simulink model "kurtosis"  (R2012b)
settings: Solver=ode45  StartTime=0.0  StopTime=3171  RelTol=1e-3
libraries: xbsIndex_r4 x3174, casper_library_flow_control x64, casper_library_misc x1, simulink_xsg_bridge x1
(part 4 of 24)

== system kurtosis/multi_to_workspace_complex/to_workspace_cplx_2 ==
  X_fi2 : Inport
  c_to_ri : Subsystem
  imag_gateway : xbsIndex_r4/Gateway Out  inherit_from_input=on  hdl_port=off  timing_constraint=None  locs_specified=off  LOCs={}  UseAsDAC=off  DACChannel='1'  block_type=gatewayout
  real_gateway : xbsIndex_r4/Gateway Out  inherit_from_input=on  hdl_port=off  timing_constraint=None  locs_specified=off  LOCs={}  UseAsDAC=off  DACChannel='1'  block_type=gatewayout
  ri_to_c : RealImagToComplex
  workspace_output : ToWorkspace  VariableName=X_fi2  SampleTime=-1
  _o : Outport
  wires:
  X_fi2/1 -> c_to_ri/1(c), _o/1
  ri_to_c/1 -> workspace_output/1  "cplx"
  imag_gateway/1 -> ri_to_c/2
  real_gateway/1 -> ri_to_c/1
  c_to_ri/2(im) -> imag_gateway/1  "c_to_ri_out2"
  c_to_ri/1(re) -> real_gateway/1  "c_to_ri_out1"

== system kurtosis/multi_to_workspace_complex/to_workspace_cplx_3 ==
  X_fi3 : Inport
  c_to_ri : Subsystem
  imag_gateway : xbsIndex_r4/Gateway Out  inherit_from_input=on  hdl_port=off  timing_constraint=None  locs_specified=off  LOCs={}  UseAsDAC=off  DACChannel='1'  block_type=gatewayout
  real_gateway : xbsIndex_r4/Gateway Out  inherit_from_input=on  hdl_port=off  timing_constraint=None  locs_specified=off  LOCs={}  UseAsDAC=off  DACChannel='1'  block_type=gatewayout
  ri_to_c : RealImagToComplex
  workspace_output : ToWorkspace  VariableName=X_fi3  SampleTime=-1
  _o : Outport
  wires:
  X_fi3/1 -> c_to_ri/1(c), _o/1
  ri_to_c/1 -> workspace_output/1  "cplx"
  imag_gateway/1 -> ri_to_c/2
  real_gateway/1 -> ri_to_c/1
  c_to_ri/2(im) -> imag_gateway/1  "c_to_ri_out2"
  c_to_ri/1(re) -> real_gateway/1  "c_to_ri_out1"

== system kurtosis/multi_to_workspace_complex/to_workspace_cplx_4 ==
  X_fi4 : Inport
  c_to_ri : Subsystem
  imag_gateway : xbsIndex_r4/Gateway Out  inherit_from_input=on  hdl_port=off  timing_constraint=None  locs_specified=off  LOCs={}  UseAsDAC=off  DACChannel='1'  block_type=gatewayout
  real_gateway : xbsIndex_r4/Gateway Out  inherit_from_input=on  hdl_port=off  timing_constraint=None  locs_specified=off  LOCs={}  UseAsDAC=off  DACChannel='1'  block_type=gatewayout
  ri_to_c : RealImagToComplex
  workspace_output : ToWorkspace  VariableName=X_fi4  SampleTime=-1
  _o : Outport
  wires:
  X_fi4/1 -> c_to_ri/1(c), _o/1
  ri_to_c/1 -> workspace_output/1  "cplx"
  imag_gateway/1 -> ri_to_c/2
  real_gateway/1 -> ri_to_c/1
  c_to_ri/2(im) -> imag_gateway/1  "c_to_ri_out2"
  c_to_ri/1(re) -> real_gateway/1  "c_to_ri_out1"

== system kurtosis/multi_to_workspace_complex/to_workspace_cplx_5 ==
  X_fi5 : Inport
  c_to_ri : Subsystem
  imag_gateway : xbsIndex_r4/Gateway Out  inherit_from_input=on  hdl_port=off  timing_constraint=None  locs_specified=off  LOCs={}  UseAsDAC=off  DACChannel='1'  block_type=gatewayout
  real_gateway : xbsIndex_r4/Gateway Out  inherit_from_input=on  hdl_port=off  timing_constraint=None  locs_specified=off  LOCs={}  UseAsDAC=off  DACChannel='1'  block_type=gatewayout
  ri_to_c : RealImagToComplex
  workspace_output : ToWorkspace  VariableName=X_fi5  SampleTime=-1
  _o : Outport
  wires:
  X_fi5/1 -> c_to_ri/1(c), _o/1
  ri_to_c/1 -> workspace_output/1  "cplx"
  imag_gateway/1 -> ri_to_c/2
  real_gateway/1 -> ri_to_c/1
  c_to_ri/2(im) -> imag_gateway/1  "c_to_ri_out2"
  c_to_ri/1(re) -> real_gateway/1  "c_to_ri_out1"

== system kurtosis/multi_to_workspace_complex/to_workspace_cplx_6 ==
  X_fi6 : Inport
  c_to_ri : Subsystem
  imag_gateway : xbsIndex_r4/Gateway Out  inherit_from_input=on  hdl_port=off  timing_constraint=None  locs_specified=off  LOCs={}  UseAsDAC=off  DACChannel='1'  block_type=gatewayout
  real_gateway : xbsIndex_r4/Gateway Out  inherit_from_input=on  hdl_port=off  timing_constraint=None  locs_specified=off  LOCs={}  UseAsDAC=off  DACChannel='1'  block_type=gatewayout
  ri_to_c : RealImagToComplex
  workspace_output : ToWorkspace  VariableName=X_fi6  SampleTime=-1
  _o : Outport
  wires:
  X_fi6/1 -> c_to_ri/1(c), _o/1
  ri_to_c/1 -> workspace_output/1  "cplx"
  imag_gateway/1 -> ri_to_c/2
  real_gateway/1 -> ri_to_c/1
  c_to_ri/2(im) -> imag_gateway/1  "c_to_ri_out2"
  c_to_ri/1(re) -> real_gateway/1  "c_to_ri_out1"

== system kurtosis/multi_to_workspace_complex/to_workspace_cplx_7 ==
  X_fi7 : Inport
  c_to_ri : Subsystem
  imag_gateway : xbsIndex_r4/Gateway Out  inherit_from_input=on  hdl_port=off  timing_constraint=None  locs_specified=off  LOCs={}  UseAsDAC=off  DACChannel='1'  block_type=gatewayout
  real_gateway : xbsIndex_r4/Gateway Out  inherit_from_input=on  hdl_port=off  timing_constraint=None  locs_specified=off  LOCs={}  UseAsDAC=off  DACChannel='1'  block_type=gatewayout
  ri_to_c : RealImagToComplex
  workspace_output : ToWorkspace  VariableName=X_fi7  SampleTime=-1
  _o : Outport
  wires:
  X_fi7/1 -> c_to_ri/1(c), _o/1
  ri_to_c/1 -> workspace_output/1  "cplx"
  imag_gateway/1 -> ri_to_c/2
  real_gateway/1 -> ri_to_c/1
  c_to_ri/2(im) -> imag_gateway/1  "c_to_ri_out2"
  c_to_ri/1(re) -> real_gateway/1  "c_to_ri_out1"

== system kurtosis/multi_to_workspace_complex/to_workspace_cplx_8 ==
  X_fi8 : Inport
  c_to_ri : Subsystem
  imag_gateway : xbsIndex_r4/Gateway Out  inherit_from_input=on  hdl_port=off  timing_constraint=None  locs_specified=off  LOCs={}  UseAsDAC=off  DACChannel='1'  block_type=gatewayout
  real_gateway : xbsIndex_r4/Gateway Out  inherit_from_input=on  hdl_port=off  timing_constraint=None  locs_specified=off  LOCs={}  UseAsDAC=off  DACChannel='1'  block_type=gatewayout
  ri_to_c : RealImagToComplex
  workspace_output : ToWorkspace  VariableName=X_fi8  SampleTime=-1
  _o : Outport
  wires:
  X_fi8/1 -> c_to_ri/1(c), _o/1
  ri_to_c/1 -> workspace_output/1  "cplx"
  imag_gateway/1 -> ri_to_c/2
  real_gateway/1 -> ri_to_c/1
  c_to_ri/2(im) -> imag_gateway/1  "c_to_ri_out2"
  c_to_ri/1(re) -> real_gateway/1  "c_to_ri_out1"

== system kurtosis/kurtosis/absx_4th_im_ser/par_to_ser ==
  pin : Inport
  ld : Inport  Port=2
  shift : Inport  Port=3
  Logical : xbsIndex_r4/Logical  logical_function=OR  inputs=2  en=off  latency=0  precision=Full  arith_type=Unsigned  n_bits=16  bin_pt=0  align_bp=on  dbl_ovrd=off  block_type=logical
  filler : xbsIndex_r4/Constant  const=0  gui_display_data_type=Fixed-point  arith_type=Unsigned  n_bits=sout_width  bin_pt=0  preci_type=Single  exp_width=8  frac_width=24  explicit_period=on  period=1  equ=P=C  opselect=C  inp2=PCIN>>17  opr=+  inp1=P  carry=CIN  dbl_ovrd=off  block_type=constant
  shifter_unit1 : casper_library_flow_control/shifter_unit  data_width=84  pin_offset=0
  shifter_unit2 : casper_library_flow_control/shifter_unit  data_width=84  pin_offset=84
  shifter_unit3 : casper_library_flow_control/shifter_unit  data_width=84  pin_offset=168
  shifter_unit4 : casper_library_flow_control/shifter_unit  data_width=84  pin_offset=252
  shifter_unit5 : casper_library_flow_control/shifter_unit  data_width=84  pin_offset=336
  shifter_unit6 : casper_library_flow_control/shifter_unit  data_width=84  pin_offset=420
  shifter_unit7 : casper_library_flow_control/shifter_unit  data_width=84  pin_offset=504
  shifter_unit8 : casper_library_flow_control/shifter_unit  data_width=84  pin_offset=588
  sout : Outport
  wires:
  ld/1 -> Logical/1, shifter_unit1/1, shifter_unit2/1, shifter_unit3/1, shifter_unit4/1, shifter_unit5/1, shifter_unit6/1, shifter_unit7/1, shifter_unit8/1
  shift/1 -> Logical/2
  filler/1 -> shifter_unit1/2
  pin/1 -> shifter_unit1/3, shifter_unit2/3, shifter_unit3/3, shifter_unit4/3, shifter_unit5/3, shifter_unit6/3, shifter_unit7/3, shifter_unit8/3
  Logical/1 -> shifter_unit1/4, shifter_unit2/4, shifter_unit3/4, shifter_unit4/4, shifter_unit5/4, shifter_unit6/4, shifter_unit7/4, shifter_unit8/4
  shifter_unit1/1 -> shifter_unit2/2
  shifter_unit2/1 -> shifter_unit3/2
  shifter_unit3/1 -> shifter_unit4/2
  shifter_unit4/1 -> shifter_unit5/2
  shifter_unit5/1 -> shifter_unit6/2
  shifter_unit6/1 -> shifter_unit7/2
  shifter_unit7/1 -> shifter_unit8/2
  shifter_unit8/1 -> sout/1

== system kurtosis/kurtosis/absx_4th_im_ser/pin_concat ==
  in0 : Inport
  in1 : Inport  Port=2
  in2 : Inport  Port=3
  in3 : Inport  Port=4
  in4 : Inport  Port=5
  in5 : Inport  Port=6
  in6 : Inport  Port=7
  in7 : Inport  Port=8
  concat : xbsIndex_r4/Concat  num_inputs=8  dbl_ovrd=off  block_type=concat
  reinterpret_{1..8} (8 alike) : xbsIndex_r4/Reinterpret  force_arith_type=on  arith_type=Unsigned  force_bin_pt=on  bin_pt=0  block_type=reinterpret
  out : Outport
  wires:
  concat/1 -> out/1
  reinterpret_8/1 -> concat/8
  reinterpret_7/1 -> concat/7
  reinterpret_6/1 -> concat/6
  reinterpret_5/1 -> concat/5
  reinterpret_4/1 -> concat/4
  reinterpret_3/1 -> concat/3
  reinterpret_2/1 -> concat/2
  reinterpret_1/1 -> concat/1
  in7/1 -> reinterpret_8/1
  in6/1 -> reinterpret_7/1
  in5/1 -> reinterpret_6/1
  in4/1 -> reinterpret_5/1
  in3/1 -> reinterpret_4/1
  in2/1 -> reinterpret_3/1
  in1/1 -> reinterpret_2/1
  in0/1 -> reinterpret_1/1

== system kurtosis/kurtosis/absx_4th_im_ser/pulse_ext ==
  ld : Inport
  Constant10 : xbsIndex_r4/Constant  const=8  gui_display_data_type=Fixed-point  arith_type=Unsigned  n_bits=4  bin_pt=0  preci_type=Single  exp_width=8  frac_width=24  explicit_period=on  period=1  equ=P=C  opselect=C  inp2=PCIN>>17  opr=+  inp1=P  carry=CIN  dbl_ovrd=off  block_type=constant
  Constant8 : xbsIndex_r4/Constant  const=15  gui_display_data_type=Fixed-point  arith_type=Unsigned  n_bits=4  bin_pt=0  preci_type=Single  exp_width=8  frac_width=24  explicit_period=on  period=1  equ=P=C  opselect=C  inp2=PCIN>>17  opr=+  inp1=P  carry=CIN  dbl_ovrd=off  block_type=constant
  Constant9 : xbsIndex_r4/Constant  const=1  gui_display_data_type=Fixed-point  arith_type=Unsigned  n_bits=4  bin_pt=0  preci_type=Single  exp_width=8  frac_width=24  explicit_period=on  period=1  equ=P=C  opselect=C  inp2=PCIN>>17  opr=+  inp1=P  carry=CIN  dbl_ovrd=off  block_type=constant
  Counter : xbsIndex_r4/Counter  cnt_type=Free Running  cnt_to=Inf  operation=Up  start_count=0  cnt_by_val=1  arith_type=Unsigned  n_bits=4  bin_pt=0  load_pin=off  rst=on  en=on  explicit_period=on  period=1  dbl_ovrd=off  use_behavioral_HDL=off  implementation=Fabric  block_type=counter
  Relational : xbsIndex_r4/Relational  mode=a<b  en=off  latency=0  dbl_ovrd=off  block_type=relational
  Relational1 : xbsIndex_r4/Relational  mode=a<=b  en=off  latency=0  dbl_ovrd=off  block_type=relational
  Relational2 : xbsIndex_r4/Relational  mode=a>=b  en=off  latency=0  dbl_ovrd=off  block_type=relational
  and : xbsIndex_r4/Logical  logical_function=AND  inputs=2  en=off  latency=0  precision=Full  arith_type=Unsigned  n_bits=16  bin_pt=0  align_bp=on  dbl_ovrd=off  block_type=logical
  or : xbsIndex_r4/Logical  logical_function=OR  inputs=2  en=off  latency=0  precision=Full  arith_type=Unsigned  n_bits=16  bin_pt=0  align_bp=on  dbl_ovrd=off  block_type=logical
  shift : Outport
  wires:
  ld/1 -> Counter/1, or/1
  Counter/1 -> Relational2/1, Relational1/1, Relational/1  "Counter_out1"
  Relational2/1 -> and/1  "Relational2_out1"
  Constant9/1 -> Relational2/2
  Relational1/1 -> and/2  "Relational1_out1"
  Constant10/1 -> Relational1/2
  Relational/1 -> or/2  "Relational_out1"
  Constant8/1 -> Relational/2
  and/1 -> shift/1
  or/1 -> Counter/2

== system kurtosis/kurtosis/absx_sq_re_ser/par_to_ser ==
  pin : Inport
  ld : Inport  Port=2
  shift : Inport  Port=3
  Logical : xbsIndex_r4/Logical  logical_function=OR  inputs=2  en=off  latency=0  precision=Full  arith_type=Unsigned  n_bits=16  bin_pt=0  align_bp=on  dbl_ovrd=off  block_type=logical
  filler : xbsIndex_r4/Constant  const=0  gui_display_data_type=Fixed-point  arith_type=Unsigned  n_bits=sout_width  bin_pt=0  preci_type=Single  exp_width=8  frac_width=24  explicit_period=on  period=1  equ=P=C  opselect=C  inp2=PCIN>>17  opr=+  inp1=P  carry=CIN  dbl_ovrd=off  block_type=constant
  shifter_unit1 : casper_library_flow_control/shifter_unit  data_width=35  pin_offset=0
  shifter_unit2 : casper_library_flow_control/shifter_unit  data_width=35  pin_offset=35
  shifter_unit3 : casper_library_flow_control/shifter_unit  data_width=35  pin_offset=70
  shifter_unit4 : casper_library_flow_control/shifter_unit  data_width=35  pin_offset=105
  shifter_unit5 : casper_library_flow_control/shifter_unit  data_width=35  pin_offset=140
  shifter_unit6 : casper_library_flow_control/shifter_unit  data_width=35  pin_offset=175
  shifter_unit7 : casper_library_flow_control/shifter_unit  data_width=35  pin_offset=210
  shifter_unit8 : casper_library_flow_control/shifter_unit  data_width=35  pin_offset=245
  sout : Outport
  wires:
  ld/1 -> Logical/1, shifter_unit1/1, shifter_unit2/1, shifter_unit3/1, shifter_unit4/1, shifter_unit5/1, shifter_unit6/1, shifter_unit7/1, shifter_unit8/1
  shift/1 -> Logical/2
  filler/1 -> shifter_unit1/2
  pin/1 -> shifter_unit1/3, shifter_unit2/3, shifter_unit3/3, shifter_unit4/3, shifter_unit5/3, shifter_unit6/3, shifter_unit7/3, shifter_unit8/3
  Logical/1 -> shifter_unit1/4, shifter_unit2/4, shifter_unit3/4, shifter_unit4/4, shifter_unit5/4, shifter_unit6/4, shifter_unit7/4, shifter_unit8/4
  shifter_unit1/1 -> shifter_unit2/2
  shifter_unit2/1 -> shifter_unit3/2
  shifter_unit3/1 -> shifter_unit4/2
  shifter_unit4/1 -> shifter_unit5/2
  shifter_unit5/1 -> shifter_unit6/2
  shifter_unit6/1 -> shifter_unit7/2
  shifter_unit7/1 -> shifter_unit8/2
  shifter_unit8/1 -> sout/1

== system kurtosis/kurtosis/absx_sq_re_ser/pin_concat ==
  in0 : Inport
  in1 : Inport  Port=2
  in2 : Inport  Port=3
  in3 : Inport  Port=4
  in4 : Inport  Port=5
  in5 : Inport  Port=6
  in6 : Inport  Port=7
  in7 : Inport  Port=8
  concat : xbsIndex_r4/Concat  num_inputs=8  dbl_ovrd=off  block_type=concat
  reinterpret_{1..8} (8 alike) : xbsIndex_r4/Reinterpret  force_arith_type=on  arith_type=Unsigned  force_bin_pt=on  bin_pt=0  block_type=reinterpret
  out : Outport
  wires:
  concat/1 -> out/1
  reinterpret_8/1 -> concat/8
  reinterpret_7/1 -> concat/7
  reinterpret_6/1 -> concat/6
  reinterpret_5/1 -> concat/5
  reinterpret_4/1 -> concat/4
  reinterpret_3/1 -> concat/3
  reinterpret_2/1 -> concat/2
  reinterpret_1/1 -> concat/1
  in7/1 -> reinterpret_8/1
  in6/1 -> reinterpret_7/1
  in5/1 -> reinterpret_6/1
  in4/1 -> reinterpret_5/1
  in3/1 -> reinterpret_4/1
  in2/1 -> reinterpret_3/1
  in1/1 -> reinterpret_2/1
  in0/1 -> reinterpret_1/1

== system kurtosis/kurtosis/absx_sq_re_ser/pulse_ext ==
  ld : Inport
  Constant10 : xbsIndex_r4/Constant  const=8  gui_display_data_type=Fixed-point  arith_type=Unsigned  n_bits=4  bin_pt=0  preci_type=Single  exp_width=8  frac_width=24  explicit_period=on  period=1  equ=P=C  opselect=C  inp2=PCIN>>17  opr=+  inp1=P  carry=CIN  dbl_ovrd=off  block_type=constant
  Constant8 : xbsIndex_r4/Constant  const=15  gui_display_data_type=Fixed-point  arith_type=Unsigned  n_bits=4  bin_pt=0  preci_type=Single  exp_width=8  frac_width=24  explicit_period=on  period=1  equ=P=C  opselect=C  inp2=PCIN>>17  opr=+  inp1=P  carry=CIN  dbl_ovrd=off  block_type=constant
  Constant9 : xbsIndex_r4/Constant  const=1  gui_display_data_type=Fixed-point  arith_type=Unsigned  n_bits=4  bin_pt=0  preci_type=Single  exp_width=8  frac_width=24  explicit_period=on  period=1  equ=P=C  opselect=C  inp2=PCIN>>17  opr=+  inp1=P  carry=CIN  dbl_ovrd=off  block_type=constant
  Counter : xbsIndex_r4/Counter  cnt_type=Free Running  cnt_to=Inf  operation=Up  start_count=0  cnt_by_val=1  arith_type=Unsigned  n_bits=4  bin_pt=0  load_pin=off  rst=on  en=on  explicit_period=on  period=1  dbl_ovrd=off  use_behavioral_HDL=off  implementation=Fabric  block_type=counter
  Relational : xbsIndex_r4/Relational  mode=a<b  en=off  latency=0  dbl_ovrd=off  block_type=relational
  Relational1 : xbsIndex_r4/Relational  mode=a<=b  en=off  latency=0  dbl_ovrd=off  block_type=relational
  Relational2 : xbsIndex_r4/Relational  mode=a>=b  en=off  latency=0  dbl_ovrd=off  block_type=relational
  and : xbsIndex_r4/Logical  logical_function=AND  inputs=2  en=off  latency=0  precision=Full  arith_type=Unsigned  n_bits=16  bin_pt=0  align_bp=on  dbl_ovrd=off  block_type=logical
  or : xbsIndex_r4/Logical  logical_function=OR  inputs=2  en=off  latency=0  precision=Full  arith_type=Unsigned  n_bits=16  bin_pt=0  align_bp=on  dbl_ovrd=off  block_type=logical
  shift : Outport
  wires:
  ld/1 -> Counter/1, or/1
  Counter/1 -> Relational2/1, Relational1/1, Relational/1  "Counter_out1"
  Relational2/1 -> and/1  "Relational2_out1"
  Constant9/1 -> Relational2/2
  Relational1/1 -> and/2  "Relational1_out1"
  Constant10/1 -> Relational1/2
  Relational/1 -> or/2  "Relational_out1"
  Constant8/1 -> Relational/2
  and/1 -> shift/1
  or/1 -> Counter/2

== system kurtosis/kurtosis/kurtosis_acc_bank_1/abs_x_4th_acc ==
  sync : Inport
  b : Inport  Port=2
  Convert : xbsIndex_r4/Convert  gui_display_data_type=Fixed-point  arith_type="Signed  (2's comp)"  n_bits=96  bin_pt=68  float_type=Single  exp_bits=8  fraction_bits=24  quantization=Truncate  overflow=Wrap  en=off  latency=0  dbl_ovrd=off  pipeline=off  block_type=convert
  DSP48E_0 : xbsIndex_r4/DSP48E  use_a=Direct from A Port  use_b=Direct from B Port  reset_preg=off  pattern_from_creg=on  pattern='000000000000'  mask_from_creg=on  pattern_mask='000000000000'  sel_rounding_mask=Select mask  use_op=off  use_creg=on  rst_all=off  en_all=off  use_pcin=off  use_carrycascin=off  use_multsignin=off  use_carryout=on  use_patterndetect=off  use_patternbdetect=off  use_overflow=off  use_underflow=off  use_acout=off  use_bcout=off  use_pcout=off  use_multsignout=off  use_carrycascout=off  pipeline_a=1  pipeline_b=1  pipeline_acout=1  pipeline_bcout=1  pipeline_c=on  pipeline_p=on  pipeline_mult=on  pipeline_opmode=on  pipeline_alumode=on  pipeline_carryin=on  pipeline_carryinsel=on  rst_a=off  rst_b=off  rst_c=off  rst_mult=off  rst_p=off  rst_carry_in=off  rst_alumode=off  rst_ctrl=off  en_a1=off  en_a2=off  en_b1=off  en_b2=off  en_c=off  en_mult=off  en_p=off  en_carry_in=off  en_alumode=off  en_multcarryin=off  en_ctrl=off  use_synth_model=off  addsub_mode=ONE48  xl_useadderonly=off  block_type=dsp48e
  DSP48E_1 : xbsIndex_r4/DSP48E  use_a=Direct from A Port  use_b=Direct from B Port  reset_preg=off  pattern_from_creg=on  pattern='000000000000'  mask_from_creg=on  pattern_mask='000000000000'  sel_rounding_mask=Select mask  use_op=off  use_creg=off  rst_all=off  en_all=off  use_pcin=off  use_carrycascin=off  use_multsignin=off  use_carryout=off  use_patterndetect=off  use_patternbdetect=off  use_overflow=off  use_underflow=off  use_acout=off  use_bcout=off  use_pcout=off  use_multsignout=off  use_carrycascout=off  pipeline_a=2  pipeline_b=2  pipeline_acout=1  pipeline_bcout=1  pipeline_c=on  pipeline_p=on  pipeline_mult=on  pipeline_opmode=on  pipeline_alumode=on  pipeline_carryin=off  pipeline_carryinsel=on  rst_a=off  rst_b=off  rst_c=off  rst_mult=off  rst_p=off  rst_carry_in=off  rst_alumode=off  rst_ctrl=off  en_a1=off  en_a2=off  en_b1=off  en_b2=off  en_c=off  en_mult=off  en_p=off  en_carry_in=off  en_alumode=off  en_multcarryin=off  en_ctrl=off  use_synth_model=off  addsub_mode=ONE48  xl_useadderonly=off  block_type=dsp48e
  DSP48_AB_splitter1 : Subsystem
  DSP48_AB_splitter2_sub : Subsystem
  Delay1 : xbsIndex_r4/Delay  rst=off  infoeditControl=Selection of Reset will increase slice count due to use of real FFs and instead of SRLs  en=off  latency=1  dbl_ovrd=off  reg_retiming=off  block_type=delay
  Mux : xbsIndex_r4/Mux  inputs=2  en=off  latency=0  precision=Full  arith_type=Unsigned  n_bits=16  bin_pt=14  quantization=Truncate  overflow=Wrap  dbl_ovrd=off  block_type=mux
  Mux1 : xbsIndex_r4/Mux  inputs=2  en=off  latency=0  precision=Full  arith_type=Unsigned  n_bits=16  bin_pt=14  quantization=Truncate  overflow=Wrap  dbl_ovrd=off  block_type=mux
  Register : xbsIndex_r4/Register  init=0  rst=off  en=off  dbl_ovrd=off  block_type=register
  Reinterpret : xbsIndex_r4/Reinterpret  force_arith_type=on  arith_type="Signed  (2's comp)"  force_bin_pt=on  bin_pt=0  block_type=reinterpret
  Reinterpret1 : xbsIndex_r4/Reinterpret  force_arith_type=on  arith_type="Signed  (2's comp)"  force_bin_pt=on  bin_pt=0  block_type=reinterpret
  Reinterpret2 : xbsIndex_r4/Reinterpret  force_arith_type=on  arith_type="Signed  (2's comp)"  force_bin_pt=on  bin_pt=68  block_type=reinterpret
  Slice : xbsIndex_r4/Slice  nbits=48  boolean_output=off  mode=Lower Bit Location + Width  bit1=0  base1=MSB of Input  bit0=0  base0=LSB of Input  dbl_ovrd=off  block_type=slice
  Slice2 : xbsIndex_r4/Slice  nbits=48  boolean_output=off  mode=Lower Bit Location + Width  bit1=0  base1=MSB of Input  bit0=48  base0=LSB of Input  dbl_ovrd=off  block_type=slice
  cram : Subsystem
  dsp48e_ctrl_init_xblock14 : Subsystem
  dsp48e_ctrl_init_xblock15 : Subsystem
  opmode_0_rst : xbsIndex_r4/Constant  const=12  gui_display_data_type=Fixed-point  arith_type=Unsigned  n_bits=7  bin_pt=0  preci_type=Single  exp_width=8  frac_width=24  explicit_period=on  period=1  equ=P=C  opselect=C  inp2=PCIN>>17  opr=+  inp1=P  carry=CIN  dbl_ovrd=off  block_type=constant
  opmode_1_rst : xbsIndex_r4/Constant  const=3  gui_display_data_type=Fixed-point  arith_type=Unsigned  n_bits=7  bin_pt=0  preci_type=Single  exp_width=8  frac_width=24  explicit_period=on  period=1  equ=P=C  opselect=C  inp2=PCIN>>17  opr=+  inp1=P  carry=CIN  dbl_ovrd=off  block_type=constant
  zero : xbsIndex_r4/Constant  const=0  gui_display_data_type=Fixed-point  arith_type=Signed (2's comp)  n_bits=48  bin_pt=0  preci_type=Single  exp_width=8  frac_width=24  explicit_period=on  period=1  equ=P=C  opselect=C  inp2=PCIN>>17  opr=+  inp1=P  carry=CIN  dbl_ovrd=off  block_type=constant
  +=b : Outport
  wires:
  sync/1 -> Mux1/1, Mux/1
  Reinterpret1/1 -> Slice2/1, Slice/1  "Reinterpret1_out1"
  dsp48e_ctrl_init_xblock15/4(carryinsel) -> DSP48E_1/6  "dsp48e_ctrl1_out4"
  dsp48e_ctrl_init_xblock15/2(alumode) -> DSP48E_1/4  "dsp48e_ctrl1_out2"
  dsp48e_ctrl_init_xblock15/1(opmode) -> Mux1/2  "dsp48e_ctrl1_out1"
  dsp48e_ctrl_init_xblock14/4(carryinsel) -> DSP48E_0/7  "dsp48e_ctrl0_out4"
  dsp48e_ctrl_init_xblock14/3(carryin) -> DSP48E_0/6  "dsp48e_ctrl0_out3"
  dsp48e_ctrl_init_xblock14/2(alumode) -> DSP48E_0/5  "dsp48e_ctrl0_out2"
  dsp48e_ctrl_init_xblock14/1(opmode) -> Mux/2  "dsp48e_ctrl0_out1"
  DSP48_AB_splitter2_sub/2(B) -> DSP48E_1/2  "DSP48_AB_splitter2_out2"
  DSP48_AB_splitter2_sub/1(A) -> DSP48E_1/1  "DSP48_AB_splitter2_out1"
  Slice2/1 -> DSP48_AB_splitter2_sub/1(A:B)  "Slice2_out1"
  zero/1 -> DSP48_AB_splitter1/1(A:B)  "zero_out1"
  opmode_1_rst/1 -> Mux1/3  "opmode_1_rst_out1"
  opmode_0_rst/1 -> Mux/3  "opmode_0_rst_out1"
  cram/1(Out) -> Reinterpret2/1  "cram_out1"
  Register/1 -> cram/2(In2)  "Register_out1"
  DSP48E_1/1 -> cram/1(In1)  "DSP48E_1_out1"
  Slice/1 -> Reinterpret/1  "Slice_out1"
  Reinterpret2/1 -> +=b/1
  Convert/1 -> Reinterpret1/1  "Convert_out1"
  Reinterpret/1 -> DSP48E_0/3  "Reinterpret_out1"
  DSP48E_0/1 -> Register/1  "DSP48E_0_out1"
  Mux1/1 -> Delay1/1  "Mux1_out1"
  Mux/1 -> DSP48E_0/4  "Mux_out1"
  Delay1/1 -> DSP48E_1/3  "Delay1_out1"
  DSP48_AB_splitter1/2(B) -> DSP48E_0/2  "DSP48_AB_splitter1_out2"
  DSP48_AB_splitter1/1(A) -> DSP48E_0/1  "DSP48_AB_splitter1_out1"
  DSP48E_0/2 -> DSP48E_1/5  "DSP48E_0_out2"
  b/1 -> Convert/1

== system kurtosis/kurtosis/kurtosis_acc_bank_1/abs_x_sq_acc ==
  sync : Inport
  b : Inport  Port=2
  Convert : xbsIndex_r4/Convert  gui_display_data_type=Fixed-point  arith_type="Signed  (2's comp)"  n_bits=96  bin_pt=34  float_type=Single  exp_bits=8  fraction_bits=24  quantization=Truncate  overflow=Wrap  en=off  latency=0  dbl_ovrd=off  pipeline=off  block_type=convert
  DSP48E_0 : xbsIndex_r4/DSP48E  use_a=Direct from A Port  use_b=Direct from B Port  reset_preg=off  pattern_from_creg=on  pattern='000000000000'  mask_from_creg=on  pattern_mask='000000000000'  sel_rounding_mask=Select mask  use_op=off  use_creg=on  rst_all=off  en_all=off  use_pcin=off  use_carrycascin=off  use_multsignin=off  use_carryout=on  use_patterndetect=off  use_patternbdetect=off  use_overflow=off  use_underflow=off  use_acout=off  use_bcout=off  use_pcout=off  use_multsignout=off  use_carrycascout=off  pipeline_a=1  pipeline_b=1  pipeline_acout=1  pipeline_bcout=1  pipeline_c=on  pipeline_p=on  pipeline_mult=on  pipeline_opmode=on  pipeline_alumode=on  pipeline_carryin=on  pipeline_carryinsel=on  rst_a=off  rst_b=off  rst_c=off  rst_mult=off  rst_p=off  rst_carry_in=off  rst_alumode=off  rst_ctrl=off  en_a1=off  en_a2=off  en_b1=off  en_b2=off  en_c=off  en_mult=off  en_p=off  en_carry_in=off  en_alumode=off  en_multcarryin=off  en_ctrl=off  use_synth_model=off  addsub_mode=ONE48  xl_useadderonly=off  block_type=dsp48e
  DSP48E_1 : xbsIndex_r4/DSP48E  use_a=Direct from A Port  use_b=Direct from B Port  reset_preg=off  pattern_from_creg=on  pattern='000000000000'  mask_from_creg=on  pattern_mask='000000000000'  sel_rounding_mask=Select mask  use_op=off  use_creg=off  rst_all=off  en_all=off  use_pcin=off  use_carrycascin=off  use_multsignin=off  use_carryout=off  use_patterndetect=off  use_patternbdetect=off  use_overflow=off  use_underflow=off  use_acout=off  use_bcout=off  use_pcout=off  use_multsignout=off  use_carrycascout=off  pipeline_a=2  pipeline_b=2  pipeline_acout=1  pipeline_bcout=1  pipeline_c=on  pipeline_p=on  pipeline_mult=on  pipeline_opmode=on  pipeline_alumode=on  pipeline_carryin=off  pipeline_carryinsel=on  rst_a=off  rst_b=off  rst_c=off  rst_mult=off  rst_p=off  rst_carry_in=off  rst_alumode=off  rst_ctrl=off  en_a1=off  en_a2=off  en_b1=off  en_b2=off  en_c=off  en_mult=off  en_p=off  en_carry_in=off  en_alumode=off  en_multcarryin=off  en_ctrl=off  use_synth_model=off  addsub_mode=ONE48  xl_useadderonly=off  block_type=dsp48e
  DSP48_AB_splitter1 : Subsystem
  DSP48_AB_splitter2_sub : Subsystem
  Delay1 : xbsIndex_r4/Delay  rst=off  infoeditControl=Selection of Reset will increase slice count due to use of real FFs and instead of SRLs  en=off  latency=1  dbl_ovrd=off  reg_retiming=off  block_type=delay
  Mux : xbsIndex_r4/Mux  inputs=2  en=off  latency=0  precision=Full  arith_type=Unsigned  n_bits=16  bin_pt=14  quantization=Truncate  overflow=Wrap  dbl_ovrd=off  block_type=mux
  Mux1 : xbsIndex_r4/Mux  inputs=2  en=off  latency=0  precision=Full  arith_type=Unsigned  n_bits=16  bin_pt=14  quantization=Truncate  overflow=Wrap  dbl_ovrd=off  block_type=mux
  Register : xbsIndex_r4/Register  init=0  rst=off  en=off  dbl_ovrd=off  block_type=register
  Reinterpret : xbsIndex_r4/Reinterpret  force_arith_type=on  arith_type="Signed  (2's comp)"  force_bin_pt=on  bin_pt=0  block_type=reinterpret
  Reinterpret1 : xbsIndex_r4/Reinterpret  force_arith_type=on  arith_type="Signed  (2's comp)"  force_bin_pt=on  bin_pt=0  block_type=reinterpret
  Reinterpret2 : xbsIndex_r4/Reinterpret  force_arith_type=on  arith_type="Signed  (2's comp)"  force_bin_pt=on  bin_pt=34  block_type=reinterpret
  Slice : xbsIndex_r4/Slice  nbits=48  boolean_output=off  mode=Lower Bit Location + Width  bit1=0  base1=MSB of Input  bit0=0  base0=LSB of Input  dbl_ovrd=off  block_type=slice
  Slice2 : xbsIndex_r4/Slice  nbits=48  boolean_output=off  mode=Lower Bit Location + Width  bit1=0  base1=MSB of Input  bit0=48  base0=LSB of Input  dbl_ovrd=off  block_type=slice
  cram : Subsystem
  dsp48e_ctrl_init_xblock12 : Subsystem
  dsp48e_ctrl_init_xblock13 : Subsystem
  opmode_0_rst : xbsIndex_r4/Constant  const=12  gui_display_data_type=Fixed-point  arith_type=Unsigned  n_bits=7  bin_pt=0  preci_type=Single  exp_width=8  frac_width=24  explicit_period=on  period=1  equ=P=C  opselect=C  inp2=PCIN>>17  opr=+  inp1=P  carry=CIN  dbl_ovrd=off  block_type=constant
  opmode_1_rst : xbsIndex_r4/Constant  const=3  gui_display_data_type=Fixed-point  arith_type=Unsigned  n_bits=7  bin_pt=0  preci_type=Single  exp_width=8  frac_width=24  explicit_period=on  period=1  equ=P=C  opselect=C  inp2=PCIN>>17  opr=+  inp1=P  carry=CIN  dbl_ovrd=off  block_type=constant
  zero : xbsIndex_r4/Constant  const=0  gui_display_data_type=Fixed-point  arith_type=Signed (2's comp)  n_bits=48  bin_pt=0  preci_type=Single  exp_width=8  frac_width=24  explicit_period=on  period=1  equ=P=C  opselect=C  inp2=PCIN>>17  opr=+  inp1=P  carry=CIN  dbl_ovrd=off  block_type=constant
  +=b : Outport
  wires:
  sync/1 -> Mux1/1, Mux/1
  Reinterpret1/1 -> Slice2/1, Slice/1  "Reinterpret1_out1"
  dsp48e_ctrl_init_xblock13/4(carryinsel) -> DSP48E_1/6  "dsp48e_ctrl1_out4"
  dsp48e_ctrl_init_xblock13/2(alumode) -> DSP48E_1/4  "dsp48e_ctrl1_out2"
  dsp48e_ctrl_init_xblock13/1(opmode) -> Mux1/2  "dsp48e_ctrl1_out1"
  dsp48e_ctrl_init_xblock12/4(carryinsel) -> DSP48E_0/7  "dsp48e_ctrl0_out4"
  dsp48e_ctrl_init_xblock12/3(carryin) -> DSP48E_0/6  "dsp48e_ctrl0_out3"
  dsp48e_ctrl_init_xblock12/2(alumode) -> DSP48E_0/5  "dsp48e_ctrl0_out2"
  dsp48e_ctrl_init_xblock12/1(opmode) -> Mux/2  "dsp48e_ctrl0_out1"
  DSP48_AB_splitter2_sub/2(B) -> DSP48E_1/2  "DSP48_AB_splitter2_out2"
  DSP48_AB_splitter2_sub/1(A) -> DSP48E_1/1  "DSP48_AB_splitter2_out1"
  Slice2/1 -> DSP48_AB_splitter2_sub/1(A:B)  "Slice2_out1"
  zero/1 -> DSP48_AB_splitter1/1(A:B)  "zero_out1"
  opmode_1_rst/1 -> Mux1/3  "opmode_1_rst_out1"
  opmode_0_rst/1 -> Mux/3  "opmode_0_rst_out1"
  cram/1(Out) -> Reinterpret2/1  "cram_out1"
  Register/1 -> cram/2(In2)  "Register_out1"
  DSP48E_1/1 -> cram/1(In1)  "DSP48E_1_out1"
  Slice/1 -> Reinterpret/1  "Slice_out1"
  Reinterpret2/1 -> +=b/1
  Convert/1 -> Reinterpret1/1  "Convert_out1"
  Reinterpret/1 -> DSP48E_0/3  "Reinterpret_out1"
  DSP48E_0/1 -> Register/1  "DSP48E_0_out1"
  Mux1/1 -> Delay1/1  "Mux1_out1"
  Mux/1 -> DSP48E_0/4  "Mux_out1"
  Delay1/1 -> DSP48E_1/3  "Delay1_out1"
  DSP48_AB_splitter1/2(B) -> DSP48E_0/2  "DSP48_AB_splitter1_out2"
  DSP48_AB_splitter1/1(A) -> DSP48E_0/1  "DSP48_AB_splitter1_out1"
  DSP48E_0/2 -> DSP48E_1/5  "DSP48E_0_out2"
  b/1 -> Convert/1

== system kurtosis/kurtosis/kurtosis_acc_bank_1/acc_rst ==
  sync : Inport
  Constant5 : xbsIndex_r4/Constant  const=1023  gui_display_data_type=Fixed-point  arith_type=Unsigned  n_bits=11  bin_pt=0  preci_type=Single  exp_width=8  frac_width=24  explicit_period=on  period=1  equ=P=C  opselect=C  inp2=PCIN>>17  opr=+  inp1=P  carry=CIN  dbl_ovrd=off  block_type=constant
  Counter : xbsIndex_r4/Counter  cnt_type=Free Running  cnt_to=Inf  operation=Up  start_count=0  cnt_by_val=1  arith_type=Unsigned  n_bits=10  bin_pt=0  load_pin=off  rst=on  en=off  explicit_period=on  period=1  dbl_ovrd=off  use_behavioral_HDL=off  implementation=Fabric  block_type=counter
  Logical : xbsIndex_r4/Logical  logical_function=OR  inputs=2  en=off  latency=0  precision=Full  arith_type=Unsigned  n_bits=16  bin_pt=0  align_bp=on  dbl_ovrd=off  block_type=logical
  Relational : xbsIndex_r4/Relational  mode=a=b  en=off  latency=0  dbl_ovrd=off  block_type=relational
  acc_del : xbsIndex_r4/Delay  rst=off  infoeditControl=Selection of Reset will increase slice count due to use of real FFs and instead of SRLs  en=off  latency=2  dbl_ovrd=off  reg_retiming=off  block_type=delay
  sync_del : xbsIndex_r4/Delay  rst=off  infoeditControl=Selection of Reset will increase slice count due to use of real FFs and instead of SRLs  en=off  latency=1  dbl_ovrd=off  reg_retiming=off  block_type=delay
  acc_rst : Outport
  sync_out : Outport  Port=2
  wires:
  sync/1 -> Logical/2, Counter/1
  Relational/1 -> sync_del/1, acc_del/1  "Relational_out1"
  sync_del/1 -> Logical/1  "sync_del_out1"
  acc_del/1 -> sync_out/1
  Constant5/1 -> Relational/2  "Constant5_out1"
  Counter/1 -> Relational/1  "Counter_out1"
  Logical/1 -> acc_rst/1

== system kurtosis/kurtosis/kurtosis_acc_bank_1/x_acc ==
  sync : Inport
  x : Inport  Port=2
  c_to_ri : Subsystem
  im_acc : Subsystem
  re_acc : Subsystem
  x_re_acc : Outport
  x_im_acc : Outport  Port=2
  wires:
  sync/1 -> im_acc/1(sync), re_acc/1(sync)
  im_acc/1(+=b) -> x_im_acc/1
  c_to_ri/2(im) -> im_acc/2(b)  "x_im"
  re_acc/1(+=b) -> x_re_acc/1
  c_to_ri/1(re) -> re_acc/2(b)  "x_re"
  x/1 -> c_to_ri/1(c)

== system kurtosis/kurtosis/kurtosis_acc_bank_1/x_cube_acc ==
  sync : Inport
  x : Inport  Port=2
  c_to_ri : Subsystem
  im_acc : Subsystem
  re_acc : Subsystem
  x_re_acc : Outport
  x_im_acc : Outport  Port=2
  wires:
  sync/1 -> im_acc/1(sync), re_acc/1(sync)
  im_acc/1(+=b) -> x_im_acc/1
  c_to_ri/2(im) -> im_acc/2(b)  "x_im"
  re_acc/1(+=b) -> x_re_acc/1
  c_to_ri/1(re) -> re_acc/2(b)  "x_re"
  x/1 -> c_to_ri/1(c)

== system kurtosis/kurtosis/kurtosis_acc_bank_1/x_sq_acc ==
  sync : Inport
  x : Inport  Port=2
  c_to_ri : Subsystem
  im_acc : Subsystem
  re_acc : Subsystem
  x_re_acc : Outport
  x_im_acc : Outport  Port=2
  wires:
  sync/1 -> im_acc/1(sync), re_acc/1(sync)
  im_acc/1(+=b) -> x_im_acc/1
  c_to_ri/2(im) -> im_acc/2(b)  "x_im"
  re_acc/1(+=b) -> x_re_acc/1
  c_to_ri/1(re) -> re_acc/2(b)  "x_re"
  x/1 -> c_to_ri/1(c)

== system kurtosis/kurtosis/kurtosis_acc_bank_2/abs_x_4th_acc ==
  sync : Inport
  b : Inport  Port=2
  Convert : xbsIndex_r4/Convert  gui_display_data_type=Fixed-point  arith_type="Signed  (2's comp)"  n_bits=96  bin_pt=68  float_type=Single  exp_bits=8  fraction_bits=24  quantization=Truncate  overflow=Wrap  en=off  latency=0  dbl_ovrd=off  pipeline=off  block_type=convert
  DSP48E_0 : xbsIndex_r4/DSP48E  use_a=Direct from A Port  use_b=Direct from B Port  reset_preg=off  pattern_from_creg=on  pattern='000000000000'  mask_from_creg=on  pattern_mask='000000000000'  sel_rounding_mask=Select mask  use_op=off  use_creg=on  rst_all=off  en_all=off  use_pcin=off  use_carrycascin=off  use_multsignin=off  use_carryout=on  use_patterndetect=off  use_patternbdetect=off  use_overflow=off  use_underflow=off  use_acout=off  use_bcout=off  use_pcout=off  use_multsignout=off  use_carrycascout=off  pipeline_a=1  pipeline_b=1  pipeline_acout=1  pipeline_bcout=1  pipeline_c=on  pipeline_p=on  pipeline_mult=on  pipeline_opmode=on  pipeline_alumode=on  pipeline_carryin=on  pipeline_carryinsel=on  rst_a=off  rst_b=off  rst_c=off  rst_mult=off  rst_p=off  rst_carry_in=off  rst_alumode=off  rst_ctrl=off  en_a1=off  en_a2=off  en_b1=off  en_b2=off  en_c=off  en_mult=off  en_p=off  en_carry_in=off  en_alumode=off  en_multcarryin=off  en_ctrl=off  use_synth_model=off  addsub_mode=ONE48  xl_useadderonly=off  block_type=dsp48e
  DSP48E_1 : xbsIndex_r4/DSP48E  use_a=Direct from A Port  use_b=Direct from B Port  reset_preg=off  pattern_from_creg=on  pattern='000000000000'  mask_from_creg=on  pattern_mask='000000000000'  sel_rounding_mask=Select mask  use_op=off  use_creg=off  rst_all=off  en_all=off  use_pcin=off  use_carrycascin=off  use_multsignin=off  use_carryout=off  use_patterndetect=off  use_patternbdetect=off  use_overflow=off  use_underflow=off  use_acout=off  use_bcout=off  use_pcout=off  use_multsignout=off  use_carrycascout=off  pipeline_a=2  pipeline_b=2  pipeline_acout=1  pipeline_bcout=1  pipeline_c=on  pipeline_p=on  pipeline_mult=on  pipeline_opmode=on  pipeline_alumode=on  pipeline_carryin=off  pipeline_carryinsel=on  rst_a=off  rst_b=off  rst_c=off  rst_mult=off  rst_p=off  rst_carry_in=off  rst_alumode=off  rst_ctrl=off  en_a1=off  en_a2=off  en_b1=off  en_b2=off  en_c=off  en_mult=off  en_p=off  en_carry_in=off  en_alumode=off  en_multcarryin=off  en_ctrl=off  use_synth_model=off  addsub_mode=ONE48  xl_useadderonly=off  block_type=dsp48e
  DSP48_AB_splitter1 : Subsystem
  DSP48_AB_splitter2_sub : Subsystem
  Delay1 : xbsIndex_r4/Delay  rst=off  infoeditControl=Selection of Reset will increase slice count due to use of real FFs and instead of SRLs  en=off  latency=1  dbl_ovrd=off  reg_retiming=off  block_type=delay
  Mux : xbsIndex_r4/Mux  inputs=2  en=off  latency=0  precision=Full  arith_type=Unsigned  n_bits=16  bin_pt=14  quantization=Truncate  overflow=Wrap  dbl_ovrd=off  block_type=mux
  Mux1 : xbsIndex_r4/Mux  inputs=2  en=off  latency=0  precision=Full  arith_type=Unsigned  n_bits=16  bin_pt=14  quantization=Truncate  overflow=Wrap  dbl_ovrd=off  block_type=mux
  Register : xbsIndex_r4/Register  init=0  rst=off  en=off  dbl_ovrd=off  block_type=register
  Reinterpret : xbsIndex_r4/Reinterpret  force_arith_type=on  arith_type="Signed  (2's comp)"  force_bin_pt=on  bin_pt=0  block_type=reinterpret
  Reinterpret1 : xbsIndex_r4/Reinterpret  force_arith_type=on  arith_type="Signed  (2's comp)"  force_bin_pt=on  bin_pt=0  block_type=reinterpret
  Reinterpret2 : xbsIndex_r4/Reinterpret  force_arith_type=on  arith_type="Signed  (2's comp)"  force_bin_pt=on  bin_pt=68  block_type=reinterpret
  Slice : xbsIndex_r4/Slice  nbits=48  boolean_output=off  mode=Lower Bit Location + Width  bit1=0  base1=MSB of Input  bit0=0  base0=LSB of Input  dbl_ovrd=off  block_type=slice
  Slice2 : xbsIndex_r4/Slice  nbits=48  boolean_output=off  mode=Lower Bit Location + Width  bit1=0  base1=MSB of Input  bit0=48  base0=LSB of Input  dbl_ovrd=off  block_type=slice
  cram : Subsystem
  dsp48e_ctrl_init_xblock30 : Subsystem
  dsp48e_ctrl_init_xblock31 : Subsystem
  opmode_0_rst : xbsIndex_r4/Constant  const=12  gui_display_data_type=Fixed-point  arith_type=Unsigned  n_bits=7  bin_pt=0  preci_type=Single  exp_width=8  frac_width=24  explicit_period=on  period=1  equ=P=C  opselect=C  inp2=PCIN>>17  opr=+  inp1=P  carry=CIN  dbl_ovrd=off  block_type=constant
  opmode_1_rst : xbsIndex_r4/Constant  const=3  gui_display_data_type=Fixed-point  arith_type=Unsigned  n_bits=7  bin_pt=0  preci_type=Single  exp_width=8  frac_width=24  explicit_period=on  period=1  equ=P=C  opselect=C  inp2=PCIN>>17  opr=+  inp1=P  carry=CIN  dbl_ovrd=off  block_type=constant
  zero : xbsIndex_r4/Constant  const=0  gui_display_data_type=Fixed-point  arith_type=Signed (2's comp)  n_bits=48  bin_pt=0  preci_type=Single  exp_width=8  frac_width=24  explicit_period=on  period=1  equ=P=C  opselect=C  inp2=PCIN>>17  opr=+  inp1=P  carry=CIN  dbl_ovrd=off  block_type=constant
  +=b : Outport
  wires:
  sync/1 -> Mux1/1, Mux/1
  Reinterpret1/1 -> Slice2/1, Slice/1  "Reinterpret1_out1"
  dsp48e_ctrl_init_xblock31/4(carryinsel) -> DSP48E_1/6  "dsp48e_ctrl1_out4"
  dsp48e_ctrl_init_xblock31/2(alumode) -> DSP48E_1/4  "dsp48e_ctrl1_out2"
  dsp48e_ctrl_init_xblock31/1(opmode) -> Mux1/2  "dsp48e_ctrl1_out1"
  dsp48e_ctrl_init_xblock30/4(carryinsel) -> DSP48E_0/7  "dsp48e_ctrl0_out4"
  dsp48e_ctrl_init_xblock30/3(carryin) -> DSP48E_0/6  "dsp48e_ctrl0_out3"
  dsp48e_ctrl_init_xblock30/2(alumode) -> DSP48E_0/5  "dsp48e_ctrl0_out2"
  dsp48e_ctrl_init_xblock30/1(opmode) -> Mux/2  "dsp48e_ctrl0_out1"
  DSP48_AB_splitter2_sub/2(B) -> DSP48E_1/2  "DSP48_AB_splitter2_out2"
  DSP48_AB_splitter2_sub/1(A) -> DSP48E_1/1  "DSP48_AB_splitter2_out1"
  Slice2/1 -> DSP48_AB_splitter2_sub/1(A:B)  "Slice2_out1"
  zero/1 -> DSP48_AB_splitter1/1(A:B)  "zero_out1"
  opmode_1_rst/1 -> Mux1/3  "opmode_1_rst_out1"
  opmode_0_rst/1 -> Mux/3  "opmode_0_rst_out1"
  cram/1(Out) -> Reinterpret2/1  "cram_out1"
  Register/1 -> cram/2(In2)  "Register_out1"
  DSP48E_1/1 -> cram/1(In1)  "DSP48E_1_out1"
  Slice/1 -> Reinterpret/1  "Slice_out1"
  Reinterpret2/1 -> +=b/1
  Convert/1 -> Reinterpret1/1  "Convert_out1"
  Reinterpret/1 -> DSP48E_0/3  "Reinterpret_out1"
  DSP48E_0/1 -> Register/1  "DSP48E_0_out1"
  Mux1/1 -> Delay1/1  "Mux1_out1"
  Mux/1 -> DSP48E_0/4  "Mux_out1"
  Delay1/1 -> DSP48E_1/3  "Delay1_out1"
  DSP48_AB_splitter1/2(B) -> DSP48E_0/2  "DSP48_AB_splitter1_out2"
  DSP48_AB_splitter1/1(A) -> DSP48E_0/1  "DSP48_AB_splitter1_out1"
  DSP48E_0/2 -> DSP48E_1/5  "DSP48E_0_out2"
  b/1 -> Convert/1

== system kurtosis/kurtosis/kurtosis_acc_bank_2/abs_x_sq_acc ==
  sync : Inport
  b : Inport  Port=2
  Convert : xbsIndex_r4/Convert  gui_display_data_type=Fixed-point  arith_type="Signed  (2's comp)"  n_bits=96  bin_pt=34  float_type=Single  exp_bits=8  fraction_bits=24  quantization=Truncate  overflow=Wrap  en=off  latency=0  dbl_ovrd=off  pipeline=off  block_type=convert
  DSP48E_0 : xbsIndex_r4/DSP48E  use_a=Direct from A Port  use_b=Direct from B Port  reset_preg=off  pattern_from_creg=on  pattern='000000000000'  mask_from_creg=on  pattern_mask='000000000000'  sel_rounding_mask=Select mask  use_op=off  use_creg=on  rst_all=off  en_all=off  use_pcin=off  use_carrycascin=off  use_multsignin=off  use_carryout=on  use_patterndetect=off  use_patternbdetect=off  use_overflow=off  use_underflow=off  use_acout=off  use_bcout=off  use_pcout=off  use_multsignout=off  use_carrycascout=off  pipeline_a=1  pipeline_b=1  pipeline_acout=1  pipeline_bcout=1  pipeline_c=on  pipeline_p=on  pipeline_mult=on  pipeline_opmode=on  pipeline_alumode=on  pipeline_carryin=on  pipeline_carryinsel=on  rst_a=off  rst_b=off  rst_c=off  rst_mult=off  rst_p=off  rst_carry_in=off  rst_alumode=off  rst_ctrl=off  en_a1=off  en_a2=off  en_b1=off  en_b2=off  en_c=off  en_mult=off  en_p=off  en_carry_in=off  en_alumode=off  en_multcarryin=off  en_ctrl=off  use_synth_model=off  addsub_mode=ONE48  xl_useadderonly=off  block_type=dsp48e
  DSP48E_1 : xbsIndex_r4/DSP48E  use_a=Direct from A Port  use_b=Direct from B Port  reset_preg=off  pattern_from_creg=on  pattern='000000000000'  mask_from_creg=on  pattern_mask='000000000000'  sel_rounding_mask=Select mask  use_op=off  use_creg=off  rst_all=off  en_all=off  use_pcin=off  use_carrycascin=off  use_multsignin=off  use_carryout=off  use_patterndetect=off  use_patternbdetect=off  use_overflow=off  use_underflow=off  use_acout=off  use_bcout=off  use_pcout=off  use_multsignout=off  use_carrycascout=off  pipeline_a=2  pipeline_b=2  pipeline_acout=1  pipeline_bcout=1  pipeline_c=on  pipeline_p=on  pipeline_mult=on  pipeline_opmode=on  pipeline_alumode=on  pipeline_carryin=off  pipeline_carryinsel=on  rst_a=off  rst_b=off  rst_c=off  rst_mult=off  rst_p=off  rst_carry_in=off  rst_alumode=off  rst_ctrl=off  en_a1=off  en_a2=off  en_b1=off  en_b2=off  en_c=off  en_mult=off  en_p=off  en_carry_in=off  en_alumode=off  en_multcarryin=off  en_ctrl=off  use_synth_model=off  addsub_mode=ONE48  xl_useadderonly=off  block_type=dsp48e
  DSP48_AB_splitter1 : Subsystem
  DSP48_AB_splitter2_sub : Subsystem
  Delay1 : xbsIndex_r4/Delay  rst=off  infoeditControl=Selection of Reset will increase slice count due to use of real FFs and instead of SRLs  en=off  latency=1  dbl_ovrd=off  reg_retiming=off  block_type=delay
  Mux : xbsIndex_r4/Mux  inputs=2  en=off  latency=0  precision=Full  arith_type=Unsigned  n_bits=16  bin_pt=14  quantization=Truncate  overflow=Wrap  dbl_ovrd=off  block_type=mux
  Mux1 : xbsIndex_r4/Mux  inputs=2  en=off  latency=0  precision=Full  arith_type=Unsigned  n_bits=16  bin_pt=14  quantization=Truncate  overflow=Wrap  dbl_ovrd=off  block_type=mux
  Register : xbsIndex_r4/Register  init=0  rst=off  en=off  dbl_ovrd=off  block_type=register
  Reinterpret : xbsIndex_r4/Reinterpret  force_arith_type=on  arith_type="Signed  (2's comp)"  force_bin_pt=on  bin_pt=0  block_type=reinterpret
  Reinterpret1 : xbsIndex_r4/Reinterpret  force_arith_type=on  arith_type="Signed  (2's comp)"  force_bin_pt=on  bin_pt=0  block_type=reinterpret
  Reinterpret2 : xbsIndex_r4/Reinterpret  force_arith_type=on  arith_type="Signed  (2's comp)"  force_bin_pt=on  bin_pt=34  block_type=reinterpret
  Slice : xbsIndex_r4/Slice  nbits=48  boolean_output=off  mode=Lower Bit Location + Width  bit1=0  base1=MSB of Input  bit0=0  base0=LSB of Input  dbl_ovrd=off  block_type=slice
  Slice2 : xbsIndex_r4/Slice  nbits=48  boolean_output=off  mode=Lower Bit Location + Width  bit1=0  base1=MSB of Input  bit0=48  base0=LSB of Input  dbl_ovrd=off  block_type=slice
  cram : Subsystem
  dsp48e_ctrl_init_xblock28 : Subsystem
  dsp48e_ctrl_init_xblock29 : Subsystem
  opmode_0_rst : xbsIndex_r4/Constant  const=12  gui_display_data_type=Fixed-point  arith_type=Unsigned  n_bits=7  bin_pt=0  preci_type=Single  exp_width=8  frac_width=24  explicit_period=on  period=1  equ=P=C  opselect=C  inp2=PCIN>>17  opr=+  inp1=P  carry=CIN  dbl_ovrd=off  block_type=constant
  opmode_1_rst : xbsIndex_r4/Constant  const=3  gui_display_data_type=Fixed-point  arith_type=Unsigned  n_bits=7  bin_pt=0  preci_type=Single  exp_width=8  frac_width=24  explicit_period=on  period=1  equ=P=C  opselect=C  inp2=PCIN>>17  opr=+  inp1=P  carry=CIN  dbl_ovrd=off  block_type=constant
  zero : xbsIndex_r4/Constant  const=0  gui_display_data_type=Fixed-point  arith_type=Signed (2's comp)  n_bits=48  bin_pt=0  preci_type=Single  exp_width=8  frac_width=24  explicit_period=on  period=1  equ=P=C  opselect=C  inp2=PCIN>>17  opr=+  inp1=P  carry=CIN  dbl_ovrd=off  block_type=constant
  +=b : Outport
  wires:
  sync/1 -> Mux1/1, Mux/1
  Reinterpret1/1 -> Slice2/1, Slice/1  "Reinterpret1_out1"
  dsp48e_ctrl_init_xblock29/4(carryinsel) -> DSP48E_1/6  "dsp48e_ctrl1_out4"
  dsp48e_ctrl_init_xblock29/2(alumode) -> DSP48E_1/4  "dsp48e_ctrl1_out2"
  dsp48e_ctrl_init_xblock29/1(opmode) -> Mux1/2  "dsp48e_ctrl1_out1"
  dsp48e_ctrl_init_xblock28/4(carryinsel) -> DSP48E_0/7  "dsp48e_ctrl0_out4"
  dsp48e_ctrl_init_xblock28/3(carryin) -> DSP48E_0/6  "dsp48e_ctrl0_out3"
  dsp48e_ctrl_init_xblock28/2(alumode) -> DSP48E_0/5  "dsp48e_ctrl0_out2"
  dsp48e_ctrl_init_xblock28/1(opmode) -> Mux/2  "dsp48e_ctrl0_out1"
  DSP48_AB_splitter2_sub/2(B) -> DSP48E_1/2  "DSP48_AB_splitter2_out2"
  DSP48_AB_splitter2_sub/1(A) -> DSP48E_1/1  "DSP48_AB_splitter2_out1"
  Slice2/1 -> DSP48_AB_splitter2_sub/1(A:B)  "Slice2_out1"
  zero/1 -> DSP48_AB_splitter1/1(A:B)  "zero_out1"
  opmode_1_rst/1 -> Mux1/3  "opmode_1_rst_out1"
  opmode_0_rst/1 -> Mux/3  "opmode_0_rst_out1"
  cram/1(Out) -> Reinterpret2/1  "cram_out1"
  Register/1 -> cram/2(In2)  "Register_out1"
  DSP48E_1/1 -> cram/1(In1)  "DSP48E_1_out1"
  Slice/1 -> Reinterpret/1  "Slice_out1"
  Reinterpret2/1 -> +=b/1
  Convert/1 -> Reinterpret1/1  "Convert_out1"
  Reinterpret/1 -> DSP48E_0/3  "Reinterpret_out1"
  DSP48E_0/1 -> Register/1  "DSP48E_0_out1"
  Mux1/1 -> Delay1/1  "Mux1_out1"
  Mux/1 -> DSP48E_0/4  "Mux_out1"
  Delay1/1 -> DSP48E_1/3  "Delay1_out1"
  DSP48_AB_splitter1/2(B) -> DSP48E_0/2  "DSP48_AB_splitter1_out2"
  DSP48_AB_splitter1/1(A) -> DSP48E_0/1  "DSP48_AB_splitter1_out1"
  DSP48E_0/2 -> DSP48E_1/5  "DSP48E_0_out2"
  b/1 -> Convert/1

== system kurtosis/kurtosis/kurtosis_acc_bank_2/acc_rst ==
  sync : Inport
  Constant5 : xbsIndex_r4/Constant  const=1023  gui_display_data_type=Fixed-point  arith_type=Unsigned  n_bits=11  bin_pt=0  preci_type=Single  exp_width=8  frac_width=24  explicit_period=on  period=1  equ=P=C  opselect=C  inp2=PCIN>>17  opr=+  inp1=P  carry=CIN  dbl_ovrd=off  block_type=constant
  Counter : xbsIndex_r4/Counter  cnt_type=Free Running  cnt_to=Inf  operation=Up  start_count=0  cnt_by_val=1  arith_type=Unsigned  n_bits=10  bin_pt=0  load_pin=off  rst=on  en=off  explicit_period=on  period=1  dbl_ovrd=off  use_behavioral_HDL=off  implementation=Fabric  block_type=counter
  Logical : xbsIndex_r4/Logical  logical_function=OR  inputs=2  en=off  latency=0  precision=Full  arith_type=Unsigned  n_bits=16  bin_pt=0  align_bp=on  dbl_ovrd=off  block_type=logical
  Relational : xbsIndex_r4/Relational  mode=a=b  en=off  latency=0  dbl_ovrd=off  block_type=relational
  acc_del : xbsIndex_r4/Delay  rst=off  infoeditControl=Selection of Reset will increase slice count due to use of real FFs and instead of SRLs  en=off  latency=2  dbl_ovrd=off  reg_retiming=off  block_type=delay
  sync_del : xbsIndex_r4/Delay  rst=off  infoeditControl=Selection of Reset will increase slice count due to use of real FFs and instead of SRLs  en=off  latency=1  dbl_ovrd=off  reg_retiming=off  block_type=delay
  acc_rst : Outport
  sync_out : Outport  Port=2
  wires:
  sync/1 -> Logical/2, Counter/1
  Relational/1 -> sync_del/1, acc_del/1  "Relational_out1"
  sync_del/1 -> Logical/1  "sync_del_out1"
  acc_del/1 -> sync_out/1
  Constant5/1 -> Relational/2  "Constant5_out1"
  Counter/1 -> Relational/1  "Counter_out1"
  Logical/1 -> acc_rst/1

== system kurtosis/kurtosis/kurtosis_acc_bank_2/x_acc ==
  sync : Inport
  x : Inport  Port=2
  c_to_ri : Subsystem
  im_acc : Subsystem
  re_acc : Subsystem
  x_re_acc : Outport
  x_im_acc : Outport  Port=2
  wires:
  sync/1 -> im_acc/1(sync), re_acc/1(sync)
  im_acc/1(+=b) -> x_im_acc/1
  c_to_ri/2(im) -> im_acc/2(b)  "x_im"
  re_acc/1(+=b) -> x_re_acc/1
  c_to_ri/1(re) -> re_acc/2(b)  "x_re"
  x/1 -> c_to_ri/1(c)

== system kurtosis/kurtosis/kurtosis_acc_bank_2/x_cube_acc ==
  sync : Inport
  x : Inport  Port=2
  c_to_ri : Subsystem
  im_acc : Subsystem
  re_acc : Subsystem
  x_re_acc : Outport
  x_im_acc : Outport  Port=2
  wires:
  sync/1 -> im_acc/1(sync), re_acc/1(sync)
  im_acc/1(+=b) -> x_im_acc/1
  c_to_ri/2(im) -> im_acc/2(b)  "x_im"
  re_acc/1(+=b) -> x_re_acc/1
  c_to_ri/1(re) -> re_acc/2(b)  "x_re"
  x/1 -> c_to_ri/1(c)

== system kurtosis/kurtosis/kurtosis_acc_bank_2/x_sq_acc ==
  sync : Inport
  x : Inport  Port=2
  c_to_ri : Subsystem
  im_acc : Subsystem
  re_acc : Subsystem
  x_re_acc : Outport
  x_im_acc : Outport  Port=2
  wires:
  sync/1 -> im_acc/1(sync), re_acc/1(sync)
  im_acc/1(+=b) -> x_im_acc/1
  c_to_ri/2(im) -> im_acc/2(b)  "x_im"
  re_acc/1(+=b) -> x_re_acc/1
  c_to_ri/1(re) -> re_acc/2(b)  "x_re"
  x/1 -> c_to_ri/1(c)
